simulink model "SD2231_Lab1_2022"  (R2020b)
settings: Solver=VariableStepAuto  StartTime=0.0  StopTime=inf  RelTol=1e-3
values from neighbouring files (symbols this model uses):
  delay = 250    [initial.m]
  K_awup = Ki_br_r/Kp_br_r    (= 10.4166666667)    [initial.m]
  K_brake = K_brake(3)    [initial.m]
  K_em = K_em(3)    [initial.m]
  Kd_br_f = 0*0.6*T_new_rl_b    (= 0)    [initial.m]
  Kd_br_r = 0.6*T_new_rl_b    (= 0.1722)    [initial.m]
  Kd_tr = 0.6*T_new    (= 0.0093)    [initial.m]
  Ki_br_f = 0.5*0.6*T_new_rl_b/L_new_rl_b^2    (= 37.3697916667)    [initial.m]
  Ki_br_r = 0.6*T_new_rl_b/L_new_rl_b^2    (= 74.7395833333)    [initial.m]
  Ki_tr = 0.6*T_new/L_new^2    (= 4.12188365651)    [initial.m]
  Kp_br_f = 1.2*T_new_rl_b/L_new_rl_b    (= 7.175)    [initial.m]
  Kp_br_r = 1.2*T_new_rl_b/L_new_rl_b    (= 7.175)    [initial.m]
  Kp_tr = 2.2*1.2*T_new/L_new    (= 0.861473684211)    [initial.m]
  N = 100    [initial.m]
  ref_br_f = 0.15    [initial.m]
  ref_br_r = 0.17-0.1    (= 0.07)    [initial.m]
  ref_tr = 0.06    [initial.m]
  step_time = 2    [initial.m]
  threshold_br_f = ref_br_f-0.05    (= 0.1)    [initial.m]
  threshold_br_r = ref_br_r-0.05    (= 0.02)    [initial.m]
  threshold_tc = ref_tr-0.02    (= 0.04)    [initial.m]
  vx_threshold = 1    [initial.m]
undefined symbols (not defined in the file or in its folder): DiscIntNeverNeededParam, Veh
libraries: CarMaker4SL x38, simulink x2, autolibmappedmotor x2
(part 3 of 4)

== system SD2231_Lab1_2022/CarMaker/Your ABS Controller/Activation Logic Br RR/Subsystem ==
  slip : Inport
  ref_slip : Inport  Port=2
  Brake Pedal : Inport  Port=3
  AdjBr RR : Scope
  PID1 : Subsystem
      settings: PortSchema="{\"entries\":[{\"content\":{\"sides\":[{\"content\":{\"connectorIds\":[\"In1\"]},\"type\":\"ConnectorPlacement.EquallySpacedRectSide\",\"uuid\":\"a0a678af-e4e1-4120-b7ef-0ef542f8e9cc\"},{\"content\":{\"connectorIds\":[\"Out1\"],\"side\":\"RIGHT\"},\"type\":\"ConnectorPlacement.EquallySpacedRectSide\",\"uuid\":\"903d0154-0882-4438-b528-a9d871d2aaef\"},{\"content\":{\"connectorIds\":[],\"side\":\"TOP\"},\"type\":\"ConnectorPlacement.EquallySpacedRectSide\",\"uuid\":\"cc0bbc94-fd35-44a3-99eb-327b952e9968\"},{\"content\":{\"connectorIds\":[\"In2\",\"In3\"],\"side\":\"BOTTOM\"},\"type\":\"ConnectorPlacement.EquallySpacedRectSide\",\"uuid\":\"05665a86-e33a-4510-a8ad-b2cae5a94577\"},{\"content\":{\"connectorIds\":[],\"side\":\"HIDDEN\"},\"type\":\"ConnectorPlacement.EquallySpacedRectSide\",\"uuid\":\"9e1bf206-7ec4-44f3-a0bc-dd9892acac44\"}]},\"type\":\"ConnectorPlacement.EquallySpacedConnector\",\"uuid\":\"274c0393-67a6-46bd-bc80-41d54c35eeb8\"}],\"packageUris\":[\"http://schema.mathworks.com/mf0/Connector/R2020b\"],\"version\":\"1.0\"}"
  Subtract : Sum  Inputs=+-
  AdjBr : Outport
  wires:
  Brake Pedal/1 -> PID1/3(Brake Pedal)
  Subtract/1 -> PID1/1(err)  "err_slip"
  ref_slip/1 -> Subtract/1
  slip/1 -> PID1/2(slip), Subtract/2
  PID1/1(AdjBrk) -> AdjBr/1, AdjBr RR/1  "AdjBr"

== system SD2231_Lab1_2022/CarMaker/Your ABS Controller/Activation Logic Br RR old 2/Controller ==
  slip : Inport
  ref_slip : Inport  Port=2
  Brake Pedal : Inport  Port=3
  AdjBrk RR : Scope
  PID : Subsystem
      settings: PortSchema="{\"entries\":[{\"content\":{\"sides\":[{\"content\":{\"connectorIds\":[\"In1\"]},\"type\":\"ConnectorPlacement.EquallySpacedRectSide\",\"uuid\":\"a0a678af-e4e1-4120-b7ef-0ef542f8e9cc\"},{\"content\":{\"connectorIds\":[\"Out1\"],\"side\":\"RIGHT\"},\"type\":\"ConnectorPlacement.EquallySpacedRectSide\",\"uuid\":\"903d0154-0882-4438-b528-a9d871d2aaef\"},{\"content\":{\"connectorIds\":[],\"side\":\"TOP\"},\"type\":\"ConnectorPlacement.EquallySpacedRectSide\",\"uuid\":\"cc0bbc94-fd35-44a3-99eb-327b952e9968\"},{\"content\":{\"connectorIds\":[\"In2\"],\"side\":\"BOTTOM\"},\"type\":\"ConnectorPlacement.EquallySpacedRectSide\",\"uuid\":\"05665a86-e33a-4510-a8ad-b2cae5a94577\"},{\"content\":{\"connectorIds\":[],\"side\":\"HIDDEN\"},\"type\":\"ConnectorPlacement.EquallySpacedRectSide\",\"uuid\":\"9e1bf206-7ec4-44f3-a0bc-dd9892acac44\"}]},\"type\":\"ConnectorPlacement.EquallySpacedConnector\",\"uuid\":\"274c0393-67a6-46bd-bc80-41d54c35eeb8\"}],\"packageUris\":[\"http://schema.mathworks.com/mf0/Connector/R2020b\"],\"version\":\"1.0\"}"
  Subtract : Sum  Inputs=+-
  err Br RR : Scope
  AdjThr : Outport
  wires:
  PID/1(AdjBrk) -> AdjBrk RR/1, AdjThr/1  "AdjTh"
  slip/1 -> Subtract/2
  ref_slip/1 -> Subtract/1
  Brake Pedal/1 -> PID/2(Brake Pedal)
  Subtract/1 -> err Br RR/1, PID/1(err)  "err_slip"

== system SD2231_Lab1_2022/CarMaker/Your ABS Controller/Activation Logic1/Subsystem ==
  slip : Inport
  ref_slip : Inport  Port=2
  PID : Subsystem
  Subtract : Sum  Inputs=+-
  AdjThr : Outport
  wires:
  PID/1(Out1) -> AdjThr/1  "AdjTh"
  Subtract/1 -> PID/1(err)  "err_slip"
  slip/1 -> Subtract/2
  ref_slip/1 -> Subtract/1

== system SD2231_Lab1_2022/CarMaker/Your ABS Controller/Activation Logic1/Subsystem1 ==
  slip : Inport
  ref_slip : Inport  Port=2
  y : Inport  Port=3
  Constant : Constant  Value=0
  PID : Subsystem
      settings: PortSchema="{\"entries\":[{\"content\":{\"sides\":[{\"content\":{\"connectorIds\":[\"In1\"]},\"type\":\"ConnectorPlacement.EquallySpacedRectSide\",\"uuid\":\"5f75fae0-be4e-4329-9d91-4f7d33fb87d9\"},{\"content\":{\"connectorIds\":[\"Out1\"],\"side\":\"RIGHT\"},\"type\":\"ConnectorPlacement.EquallySpacedRectSide\",\"uuid\":\"c361bfc5-4855-4965-a149-2e455cce300e\"},{\"content\":{\"connectorIds\":[],\"side\":\"TOP\"},\"type\":\"ConnectorPlacement.EquallySpacedRectSide\",\"uuid\":\"fade0fb3-5f05-4ac2-a1e9-f009226e3d9f\"},{\"content\":{\"connectorIds\":[\"In2\"],\"side\":\"BOTTOM\"},\"type\":\"ConnectorPlacement.EquallySpacedRectSide\",\"uuid\":\"3a93efea-c75a-4538-a3be-ea0ed2ce111d\"},{\"content\":{\"connectorIds\":[],\"side\":\"HIDDEN\"},\"type\":\"ConnectorPlacement.EquallySpacedRectSide\",\"uuid\":\"d2f329f2-1496-4710-b496-1fae21ed404d\"}]},\"type\":\"ConnectorPlacement.EquallySpacedConnector\",\"uuid\":\"49448e82-eaef-46f2-a659-58ee303f2511\"}],\"packageUris\":[\"http://schema.mathworks.com/mf0/Connector/R2020b\"],\"version\":\"1.0\"}"
  Subtract : Sum  Inputs=+-
  Switch : Switch  Criteria=u2 > Threshold  Threshold=0.5
  AdjThr : Outport
  wires:
  PID/1(Out1) -> AdjThr/1  "AdjTh"
  Subtract/1 -> Switch/1  "err_slip"
  ref_slip/1 -> Subtract/1
  slip/1 -> Subtract/2
  y/1 -> PID/2(y), Switch/2
  Switch/1 -> PID/1(err)
  Constant/1 -> Switch/3

== system SD2231_Lab1_2022/CarMaker/Your Traction Controller/Activation Logic RL tr1/If Action Subsystem ==
  Throttle : Inport
  Action Port : ActionPort
  Out1 : Outport
  wires:
  Throttle/1 -> Out1/1

== system SD2231_Lab1_2022/CarMaker/Your Traction Controller/Activation Logic RL tr1/Subsystem ==
  slip : Inport
  ref_slip : Inport  Port=2
  PID : Subsystem
  Subtract : Sum  Inputs=+-
  AdjThr : Outport
  wires:
  ref_slip/1 -> Subtract/1
  slip/1 -> Subtract/2
  Subtract/1 -> PID/1(err)  "err_slip"
  PID/1(Out1) -> AdjThr/1  "AdjTh"

== system SD2231_Lab1_2022/CarMaker/Your Traction Controller/Activation Logic RL tr1/Subsystem1 ==
  slip : Inport
  ref_slip : Inport  Port=2
  Thr : Inport  Port=3
  Action Port : ActionPort  InitializeStates=reset
  Add : Sum
  PID : Subsystem
  Scope : Scope
  Subtract : Sum  Inputs=+-
  AdjThr : Outport
  wires:
  slip/1 -> Subtract/2
  ref_slip/1 -> Subtract/1
  Subtract/1 -> PID/1(err)  "err_slip"
  PID/1(Out1) -> Add/1, Scope/1  "AdjTh"
  Add/1 -> AdjThr/1
  Thr/1 -> Add/2

== system SD2231_Lab1_2022/CarMaker/Your Traction Controller/Activation Logic RL tr2/Subsystem ==
  slip : Inport
  ref_slip : Inport  Port=2
  PID : Subsystem
  Subtract : Sum  Inputs=+-
  AdjThr : Outport
  wires:
  ref_slip/1 -> Subtract/1
  slip/1 -> Subtract/2
  Subtract/1 -> PID/1(err)  "err_slip"
  PID/1(Out1) -> AdjThr/1  "AdjTh"

== system SD2231_Lab1_2022/CarMaker/Your Traction Controller/Activation Logic RL tr2/Subsystem2 ==
  slip : Inport
  ref_slip : Inport  Port=2
  PID : Subsystem
  Scope : Scope
  Subtract : Sum  Inputs=+-
  AdjThr : Outport
  wires:
  PID/1(Out1) -> Scope/1, AdjThr/1  "AdjTh"
  Subtract/1 -> PID/1(err)  "err_slip"
  ref_slip/1 -> Subtract/1
  slip/1 -> Subtract/2

== system SD2231_Lab1_2022/CarMaker/Your Traction Controller/Activation Logic Tr RL/Subsystem ==
  slip : Inport
  ref_slip : Inport  Port=2
  <Throttle> : Inport  Port=3
  PID : Subsystem
      settings: PortSchema="{\"entries\":[{\"content\":{\"sides\":[{\"content\":{\"connectorIds\":[\"In1\"]},\"type\":\"ConnectorPlacement.EquallySpacedRectSide\",\"uuid\":\"27c74ca7-1daa-4fc0-829c-217569941054\"},{\"content\":{\"connectorIds\":[\"Out1\"],\"side\":\"RIGHT\"},\"type\":\"ConnectorPlacement.EquallySpacedRectSide\",\"uuid\":\"bade77b6-0597-4f1a-8de0-ed17ea00e333\"},{\"content\":{\"connectorIds\":[],\"side\":\"TOP\"},\"type\":\"ConnectorPlacement.EquallySpacedRectSide\",\"uuid\":\"4b619bdf-cd00-481e-98d9-26786e320dd0\"},{\"content\":{\"connectorIds\":[\"In2\",\"In3\"],\"side\":\"BOTTOM\"},\"type\":\"ConnectorPlacement.EquallySpacedRectSide\",\"uuid\":\"91517f3b-551d-4be5-b03a-3be9321d6908\"},{\"content\":{\"connectorIds\":[],\"side\":\"HIDDEN\"},\"type\":\"ConnectorPlacement.EquallySpacedRectSide\",\"uuid\":\"07589139-3665-4dc7-ae4e-788dbab128c2\"}]},\"type\":\"ConnectorPlacement.EquallySpacedConnector\",\"uuid\":\"e768313e-81de-4048-a761-0fa329904525\"}],\"packageUris\":[\"http://schema.mathworks.com/mf0/Connector/R2020b\"],\"version\":\"1.0\"}"
  Scope : Scope
  Subtract : Sum  Inputs=+-
  AdjThr : Outport
  wires:
  PID/1(AdjThr) -> AdjThr/1  "AdjTh"
  Subtract/1 -> Scope/1, PID/1(err)  "err_slip"
  slip/1 -> PID/2(slip), Subtract/2
  ref_slip/1 -> Subtract/1
  <Throttle>/1 -> PID/3(<Throttle>)

== system SD2231_Lab1_2022/CarMaker/Your Traction Controller/Activation Logic Tr RR/Controller ==
  slip : Inport
  ref_slip : Inport  Port=2
  Thr : Inport  Port=3
  AdjThr Tr RR : Scope
  MATLAB Function : MATLAB Function  TreatAsAtomicUnit=on
  PID : Subsystem
      settings: PortSchema="{\"entries\":[{\"content\":{\"sides\":[{\"content\":{\"connectorIds\":[\"In1\"]},\"type\":\"ConnectorPlacement.EquallySpacedRectSide\",\"uuid\":\"d5b4ba42-8bbc-455d-8ebe-912fe1a5c4b4\"},{\"content\":{\"connectorIds\":[\"Out1\"],\"side\":\"RIGHT\"},\"type\":\"ConnectorPlacement.EquallySpacedRectSide\",\"uuid\":\"23c8bac9-5734-4043-a20e-1b8e92118956\"},{\"content\":{\"connectorIds\":[\"In2\"],\"side\":\"TOP\"},\"type\":\"ConnectorPlacement.EquallySpacedRectSide\",\"uuid\":\"5c7d1d7e-636d-433e-8c10-d4c1c9edca3a\"},{\"content\":{\"connectorIds\":[],\"side\":\"HIDDEN\"},\"type\":\"ConnectorPlacement.EquallySpacedRectSide\",\"uuid\":\"05139430-708c-42b5-9da5-332763797e2c\"}]},\"type\":\"ConnectorPlacement.EquallySpacedConnector\",\"uuid\":\"3630f8de-e8d3-4428-bdc8-7dd499871779\"}],\"packageUris\":[\"http://schema.mathworks.com/mf0/Connector/R2020b\"],\"version\":\"1.0\"}"
  Subtract : Sum  Inputs=+-
  err Tr RR : Scope
  AdjThr : Outport
  wires:
  PID/1(Out1) -> AdjThr Tr RR/1, AdjThr/1  "AdjTh"
  Subtract/1 -> err Tr RR/1, PID/1(err)  "err_slip"
  slip/1 -> Subtract/2
  ref_slip/1 -> Subtract/1
  Thr/1 -> MATLAB Function/1(Brk)
  MATLAB Function/1(res) -> PID/2(res)

== system SD2231_Lab1_2022/CarMaker/Your Traction Controller/Activation Logic Tr RR/Subsystem ==
  slip : Inport
  ref_slip : Inport  Port=2
  <Throttle> : Inport  Port=3
  PID : Subsystem
      settings: PortSchema="{\"entries\":[{\"content\":{\"sides\":[{\"content\":{\"connectorIds\":[\"In1\"]},\"type\":\"ConnectorPlacement.EquallySpacedRectSide\",\"uuid\":\"27c74ca7-1daa-4fc0-829c-217569941054\"},{\"content\":{\"connectorIds\":[\"Out1\"],\"side\":\"RIGHT\"},\"type\":\"ConnectorPlacement.EquallySpacedRectSide\",\"uuid\":\"bade77b6-0597-4f1a-8de0-ed17ea00e333\"},{\"content\":{\"connectorIds\":[],\"side\":\"TOP\"},\"type\":\"ConnectorPlacement.EquallySpacedRectSide\",\"uuid\":\"4b619bdf-cd00-481e-98d9-26786e320dd0\"},{\"content\":{\"connectorIds\":[\"In2\",\"In3\"],\"side\":\"BOTTOM\"},\"type\":\"ConnectorPlacement.EquallySpacedRectSide\",\"uuid\":\"91517f3b-551d-4be5-b03a-3be9321d6908\"},{\"content\":{\"connectorIds\":[],\"side\":\"HIDDEN\"},\"type\":\"ConnectorPlacement.EquallySpacedRectSide\",\"uuid\":\"07589139-3665-4dc7-ae4e-788dbab128c2\"}]},\"type\":\"ConnectorPlacement.EquallySpacedConnector\",\"uuid\":\"e768313e-81de-4048-a761-0fa329904525\"}],\"packageUris\":[\"http://schema.mathworks.com/mf0/Connector/R2020b\"],\"version\":\"1.0\"}"
  Scope : Scope
  Subtract : Sum  Inputs=+-
  AdjThr : Outport
  wires:
  PID/1(AdjThr) -> AdjThr/1  "AdjTh"
  Subtract/1 -> Scope/1, PID/1(err)  "err_slip"
  slip/1 -> PID/2(slip), Subtract/2
  ref_slip/1 -> Subtract/1
  <Throttle>/1 -> PID/3(<Throttle>)

== system SD2231_Lab1_2022/CarMaker/Your Traction Controller/Activation Logic1/Subsystem ==
  slip : Inport
  ref_slip : Inport  Port=2
  PID : Subsystem
  Subtract : Sum  Inputs=+-
  AdjThr : Outport
  wires:
  PID/1(Out1) -> AdjThr/1  "AdjTh"
  Subtract/1 -> PID/1(err)  "err_slip"
  slip/1 -> Subtract/2
  ref_slip/1 -> Subtract/1

== system SD2231_Lab1_2022/CarMaker/Your observer/Slip observer/ FL slip subsys ==
  note: Traction Slip
  note: Braking Slip
  Vehicle velocity : Inport
  " Tyre radius" : Inport  Port=2
  Tyre rot vel : Inport  Port=3
  Divide : Product  Inputs=*/
  Divide1 : Product  Inputs=**
  Divide2 : Product  Inputs=*/
  Divide3 : Product  Inputs=**
  Saturation : Saturate  UpperLimit=inf  LowerLimit=0.5
  Saturation1 : Saturate  UpperLimit=inf  LowerLimit=0.5
  Scope : Scope  NumInputPorts=2
  Subtract1 : Sum  Inputs=-+
  Subtract2 : Sum  Inputs=+-
  trac_slip : Outport
  brak_slip : Outport  Port=2
  wires:
  Subtract2/1 -> Divide2/1  "r*w-vx"
  Subtract1/1 -> Divide/1  "r*w-vx"
  Divide2/1 -> Scope/2, brak_slip/1  "brak_slip"
  Divide/1 -> Scope/1, trac_slip/1  "trac_slip"
  Vehicle velocity/1 -> Saturation1/1, Subtract2/1, Subtract1/1
  Divide3/1 -> Subtract2/2  "r*w"
  Divide1/1 -> Saturation/1, Subtract1/2  "r*w"
  " Tyre radius"/1 -> Divide3/1, Divide1/1
  Tyre rot vel/1 -> Divide3/2, Divide1/2
  Saturation/1 -> Divide/2
  Saturation1/1 -> Divide2/2

== system SD2231_Lab1_2022/CarMaker/Your observer/Slip observer/ FR slip subsys ==
  note: Braking Slip
  note: Traction Slip
  Vehicle velocity : Inport
  " Tyre radius" : Inport  Port=2
  Tyre rot vel : Inport  Port=3
  Divide : Product  Inputs=*/
  Divide1 : Product  Inputs=**
  Divide2 : Product  Inputs=*/
  Divide3 : Product  Inputs=**
  Gain1 : Gain  Commented=on  Gain=-1
  Saturation : Saturate  UpperLimit=inf  LowerLimit=0.5
  Saturation1 : Saturate  UpperLimit=inf  LowerLimit=0.5
  Scope : Scope  NumInputPorts=2
  Subtract1 : Sum  Inputs=-+
  Subtract2 : Sum  Inputs=+-
  Switch4 : Switch  Commented=on  Criteria=u2 > Threshold
  trac_slip : Outport
  brak_slip : Outport  Port=2
  wires:
  Tyre rot vel/1 -> Divide1/2, Divide3/2
  " Tyre radius"/1 -> Divide1/1, Divide3/1
  Divide1/1 -> Saturation/1, Subtract1/2  "r*w"
  Gain1/1 -> Switch4/3
  Divide3/1 -> Subtract2/2  "r*w"
  Vehicle velocity/1 -> Subtract1/1, Saturation1/1, Subtract2/1
  Divide/1 -> trac_slip/1, Scope/1  "trac_slip"
  Divide2/1 -> brak_slip/1, Scope/2  "brak_slip"
  Subtract1/1 -> Divide/1  "r*w-vx"
  Subtract2/1 -> Divide2/1  "r*w-vx"
  Saturation/1 -> Divide/2
  Saturation1/1 -> Divide2/2

== system SD2231_Lab1_2022/CarMaker/Your observer/Slip observer/ RL slip subsys ==
  note: Braking Slip
  note: Traction Slip
  Vehicle velocity : Inport
  " Tyre radius" : Inport  Port=2
  Tyre rot vel : Inport  Port=3
  Divide : Product  Inputs=*/
  Divide1 : Product  Inputs=**
  Divide2 : Product  Inputs=*/
  Divide3 : Product  Inputs=**
  Gain1 : Gain  Commented=on  Gain=-1
  Saturation : Saturate  UpperLimit=inf  LowerLimit=0.5
  Saturation1 : Saturate  UpperLimit=inf  LowerLimit=0.5
  Scope : Scope  NumInputPorts=2
  Subtract1 : Sum  Inputs=-+
  Subtract2 : Sum  Inputs=+-
  Switch4 : Switch  Commented=on  Criteria=u2 > Threshold
  trac_slip : Outport
  brak_slip : Outport  Port=2
  wires:
  Tyre rot vel/1 -> Divide1/2, Divide3/2
  " Tyre radius"/1 -> Divide1/1, Divide3/1
  Divide1/1 -> Saturation/1, Subtract1/2  "r*w"
  Gain1/1 -> Switch4/3
  Divide3/1 -> Subtract2/2  "r*w"
  Vehicle velocity/1 -> Subtract1/1, Saturation1/1, Subtract2/1
  Divide/1 -> trac_slip/1, Scope/1  "trac_slip"
  Divide2/1 -> brak_slip/1, Scope/2  "brak_slip"
  Subtract1/1 -> Divide/1  "r*w-vx"
  Subtract2/1 -> Divide2/1  "r*w-vx"
  Saturation/1 -> Divide/2
  Saturation1/1 -> Divide2/2

== system SD2231_Lab1_2022/CarMaker/Your observer/Slip observer/ RR slip subsys ==
  note: Braking Slip
  note: Traction Slip
  Vehicle velocity : Inport
  " Tyre radius" : Inport  Port=2
  Tyre rot vel : Inport  Port=3
  Divide : Product  Inputs=*/
  Divide1 : Product  Inputs=**
  Divide2 : Product  Inputs=*/
  Divide3 : Product  Inputs=**
  Gain1 : Gain  Commented=on  Gain=-1
  Saturation : Saturate  UpperLimit=inf  LowerLimit=0.5
  Saturation1 : Saturate  UpperLimit=inf  LowerLimit=0.5
  Scope : Scope  NumInputPorts=2
  Subtract1 : Sum  Inputs=-+
  Subtract2 : Sum  Inputs=+-
  Switch4 : Switch  Commented=on  Criteria=u2 > Threshold
  trac_slip : Outport
  brak_slip : Outport  Port=2
  wires:
  Tyre rot vel/1 -> Divide1/2, Divide3/2
  " Tyre radius"/1 -> Divide1/1, Divide3/1
  Divide1/1 -> Saturation/1, Subtract1/2  "r*w"
  Gain1/1 -> Switch4/3
  Divide3/1 -> Subtract2/2  "r*w"
  Vehicle velocity/1 -> Subtract1/1, Saturation1/1, Subtract2/1
  Divide/1 -> trac_slip/1, Scope/1  "trac_slip"
  Divide2/1 -> brak_slip/1, Scope/2  "brak_slip"
  Subtract1/1 -> Divide/1  "r*w-vx"
  Subtract2/1 -> Divide2/1  "r*w-vx"
  Saturation/1 -> Divide/2
  Saturation1/1 -> Divide2/2

== system SD2231_Lab1_2022/CarMaker/IPG Vehicle/Brake/UserDefinedBrakingSystem/Subsystem ==
  FLBrakeAdjust : Inport
  BrakeFrcMax : Constant  Value=K_brake
  Gain : Gain  Gain=180.0/300.0  SaturateOnIntegerOverflow=on  OutDataTypeStr=Inherit: Same as input  ParamDataTypeStr=Inherit: Same as input
  Pedal Force : Product  InputSameDT=on  SaturateOnIntegerOverflow=on  OutDataTypeStr=Inherit: Same as first input
  Pedal Force1 : Product  InputSameDT=on  SaturateOnIntegerOverflow=on  OutDataTypeStr=Inherit: Same as first input
  pWB2Trq Front bias : Constant  Value=10
  FL brake force : Outport  VectorParamsAs1DForOutWhenUnconnected=off
  wires:
  Pedal Force/1 -> Gain/1
  BrakeFrcMax/1 -> Pedal Force/2
  Gain/1 -> Pedal Force1/1
  FLBrakeAdjust/1 -> Pedal Force/1
  pWB2Trq Front bias/1 -> Pedal Force1/2
  Pedal Force1/1 -> FL brake force/1

== system SD2231_Lab1_2022/CarMaker/IPG Vehicle/Brake/UserDefinedBrakingSystem/Subsystem1 ==
  FRBrakeAdjust : Inport
  BrakeFrcMax : Constant  Value=K_brake
  Gain : Gain  Gain=180.0/300.0  SaturateOnIntegerOverflow=on  OutDataTypeStr=Inherit: Same as input  ParamDataTypeStr=Inherit: Same as input
  Pedal Force : Product  InputSameDT=on  SaturateOnIntegerOverflow=on  OutDataTypeStr=Inherit: Same as first input
  Pedal Force1 : Product  InputSameDT=on  SaturateOnIntegerOverflow=on  OutDataTypeStr=Inherit: Same as first input
  pWB2Trq Front bias : Constant  Value=10
  FR brake force : Outport  VectorParamsAs1DForOutWhenUnconnected=off
  wires:
  Pedal Force/1 -> Gain/1
  BrakeFrcMax/1 -> Pedal Force/2
  Gain/1 -> Pedal Force1/1
  FRBrakeAdjust/1 -> Pedal Force/1
  pWB2Trq Front bias/1 -> Pedal Force1/2
  Pedal Force1/1 -> FR brake force/1

== system SD2231_Lab1_2022/CarMaker/IPG Vehicle/Brake/UserDefinedBrakingSystem/Subsystem2 ==
  RLBrakeAdjust : Inport
  BrakeFrcMax : Constant  Value=K_brake
  Gain : Gain  Gain=180.0/300.0  SaturateOnIntegerOverflow=on  OutDataTypeStr=Inherit: Same as input  ParamDataTypeStr=Inherit: Same as input
  Pedal Force : Product  InputSameDT=on  SaturateOnIntegerOverflow=on  OutDataTypeStr=Inherit: Same as first input
  Pedal Force1 : Product  InputSameDT=on  SaturateOnIntegerOverflow=on  OutDataTypeStr=Inherit: Same as first input
  pWB2Trq Rear bias : Constant  Value=4
  RL brake force : Outport  VectorParamsAs1DForOutWhenUnconnected=off
  wires:
  Pedal Force/1 -> Gain/1
  BrakeFrcMax/1 -> Pedal Force/2
  Gain/1 -> Pedal Force1/1
  RLBrakeAdjust/1 -> Pedal Force/1
  pWB2Trq Rear bias/1 -> Pedal Force1/2
  Pedal Force1/1 -> RL brake force/1

== system SD2231_Lab1_2022/CarMaker/IPG Vehicle/Brake/UserDefinedBrakingSystem/Subsystem3 ==
  RRBrakeAdjust : Inport
  BrakeFrcMax : Constant  Value=K_brake
  Gain : Gain  Gain=180.0/300.0  SaturateOnIntegerOverflow=on  OutDataTypeStr=Inherit: Same as input  ParamDataTypeStr=Inherit: Same as input
  Pedal Force : Product  InputSameDT=on  SaturateOnIntegerOverflow=on  OutDataTypeStr=Inherit: Same as first input
  Pedal Force1 : Product  InputSameDT=on  SaturateOnIntegerOverflow=on  OutDataTypeStr=Inherit: Same as first input
  pWB2Trq Rear bias : Constant  Value=4
  RR brake force : Outport  VectorParamsAs1DForOutWhenUnconnected=off
  wires:
  Pedal Force/1 -> Gain/1
  BrakeFrcMax/1 -> Pedal Force/2
  Gain/1 -> Pedal Force1/1
  RRBrakeAdjust/1 -> Pedal Force/1
  pWB2Trq Rear bias/1 -> Pedal Force1/2
  Pedal Force1/1 -> RR brake force/1

== system SD2231_Lab1_2022/CarMaker/IPG Vehicle/CarAndTrailer/CarAndTrailerUpd/CreateBus Brake.IF.In ==
  In : Inport
  BusCreator : BusCreator  Inputs=9
  Demux : Demux  Outputs=9
      settings: DisplayOption=none
  Out : Outport
  wires:
  Demux/9 -> BusCreator/9  "Brake IF Trq_Reg RR"
  Demux/8 -> BusCreator/8  "Brake IF Trq_Reg RL"
  Demux/7 -> BusCreator/7  "Brake IF Trq_Reg FR"
  Demux/6 -> BusCreator/6  "Brake IF Trq_Reg FL"
  Demux/5 -> BusCreator/5  "Brake IF Trq_Reg_max RR"
  Demux/4 -> BusCreator/4  "Brake IF Trq_Reg_max RL"
  Demux/3 -> BusCreator/3  "Brake IF Trq_Reg_max FR"
  Demux/2 -> BusCreator/2  "Brake IF Trq_Reg_max FL"
  Demux/1 -> BusCreator/1  "Brake IF T_env"
  BusCreator/1 -> Out/1
  In/1 -> Demux/1

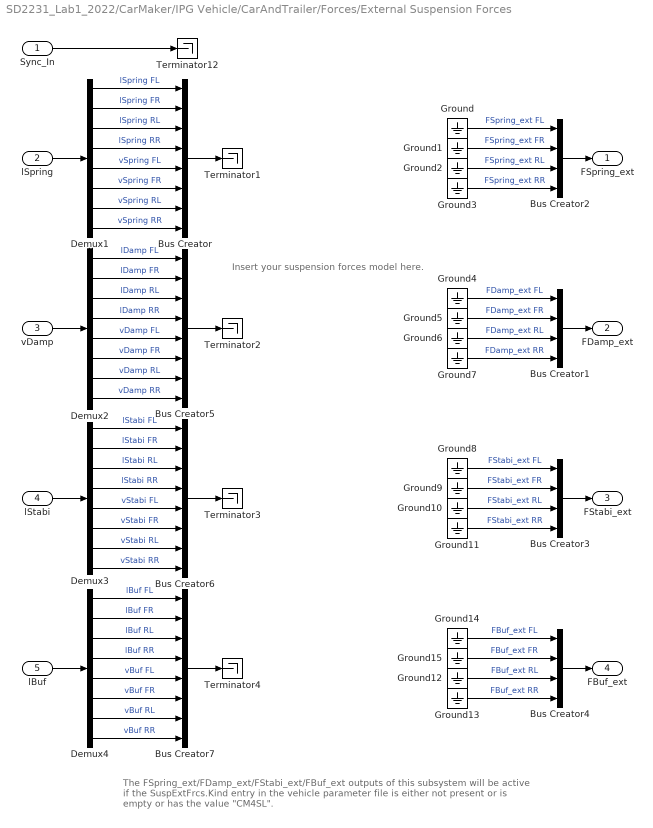
== system SD2231_Lab1_2022/CarMaker/IPG Vehicle/CarAndTrailer/Forces/External Suspension Forces ==
  note: The FSpring_ext/FDamp_ext/FStabi_ext/FBuf_ext outputs of this subsystem will be
      | active if the SuspExtFrcs.Kind entry in the vehicle parameter file
      | is either not present or is empty or has the value "CM4SL".
  note: Insert your suspension forces model here.
  Sync_In : Inport
  lSpring : Inport  Port=2
  vDamp : Inport  Port=3
  lStabi : Inport  Port=4
  lBuf : Inport  Port=5
  Bus Creator{,5..7} (4 alike) : BusCreator  Inputs=8
  Bus Creator{1..4} (4 alike) : BusCreator  Inputs=4
  Demux{1..4} (4 alike) : Demux  Outputs=8
      settings: DisplayOption=none
  Ground{,1..15} (16 alike) : Ground
  Terminator{1..4,12} (5 alike) : Terminator
  FSpring_ext : Outport
  FDamp_ext : Outport  Port=2
  FStabi_ext : Outport  Port=3
  FBuf_ext : Outport  Port=4
  wires:
  Bus Creator7/1 -> Terminator4/1
  Bus Creator6/1 -> Terminator3/1
  Bus Creator5/1 -> Terminator2/1
  Bus Creator/1 -> Terminator1/1
  Demux4/8 -> Bus Creator7/8  "vBuf RR"
  Demux4/7 -> Bus Creator7/7  "vBuf RL"
  Demux4/6 -> Bus Creator7/6  "vBuf FR"
  Demux4/5 -> Bus Creator7/5  "vBuf FL"
  Demux3/8 -> Bus Creator6/8  "vStabi RR"
  Demux3/7 -> Bus Creator6/7  "vStabi RL"
  Demux3/6 -> Bus Creator6/6  "vStabi FR"
  Demux3/5 -> Bus Creator6/5  "vStabi FL"
  Demux2/8 -> Bus Creator5/8  "vDamp RR"
  Demux2/7 -> Bus Creator5/7  "vDamp RL"
  Demux2/6 -> Bus Creator5/6  "vDamp FR"
  Demux2/5 -> Bus Creator5/5  "vDamp FL"
  Demux1/8 -> Bus Creator/8  "vSpring RR"
  Demux1/7 -> Bus Creator/7  "vSpring RL"
  Demux1/6 -> Bus Creator/6  "vSpring FR"
  Demux1/5 -> Bus Creator/5  "vSpring FL"
  Demux2/4 -> Bus Creator5/4  "lDamp RR"
  Demux2/3 -> Bus Creator5/3  "lDamp RL"
  Demux2/2 -> Bus Creator5/2  "lDamp FR"
  Demux2/1 -> Bus Creator5/1  "lDamp FL"
  Demux1/4 -> Bus Creator/4  "lSpring RR"
  Demux1/3 -> Bus Creator/3  "lSpring RL"
  Demux1/2 -> Bus Creator/2  "lSpring FR"
  Demux1/1 -> Bus Creator/1  "lSpring FL"
  Demux3/4 -> Bus Creator6/4  "lStabi RR"
  Demux3/3 -> Bus Creator6/3  "lStabi RL"
  Demux3/2 -> Bus Creator6/2  "lStabi FR"
  Demux3/1 -> Bus Creator6/1  "lStabi FL"
  lStabi/1 -> Demux3/1
  vDamp/1 -> Demux2/1
  lSpring/1 -> Demux1/1
  Demux4/4 -> Bus Creator7/4  "lBuf RR"
  Demux4/3 -> Bus Creator7/3  "lBuf RL"
  Demux4/2 -> Bus Creator7/2  "lBuf FR"
  Demux4/1 -> Bus Creator7/1  "lBuf FL"
  lBuf/1 -> Demux4/1
  Ground14/1 -> Bus Creator4/1  "FBuf_ext FL"
  Ground15/1 -> Bus Creator4/2  "FBuf_ext FR"
  Ground12/1 -> Bus Creator4/3  "FBuf_ext RL"
  Ground13/1 -> Bus Creator4/4  "FBuf_ext RR"
  Bus Creator4/1 -> FBuf_ext/1
  Sync_In/1 -> Terminator12/1
  Bus Creator2/1 -> FSpring_ext/1
  Ground/1 -> Bus Creator2/1  "FSpring_ext FL"
  Ground1/1 -> Bus Creator2/2  "FSpring_ext FR"
  Ground2/1 -> Bus Creator2/3  "FSpring_ext RL"
  Ground3/1 -> Bus Creator2/4  "FSpring_ext RR"
  Ground4/1 -> Bus Creator1/1  "FDamp_ext FL"
  Ground5/1 -> Bus Creator1/2  "FDamp_ext FR"
  Ground6/1 -> Bus Creator1/3  "FDamp_ext RL"
  Ground7/1 -> Bus Creator1/4  "FDamp_ext RR"
  Bus Creator1/1 -> FDamp_ext/1
  Ground8/1 -> Bus Creator3/1  "FStabi_ext FL"
  Ground9/1 -> Bus Creator3/2  "FStabi_ext FR"
  Ground10/1 -> Bus Creator3/3  "FStabi_ext RL"
  Ground11/1 -> Bus Creator3/4  "FStabi_ext RR"
  Bus Creator3/1 -> FStabi_ext/1

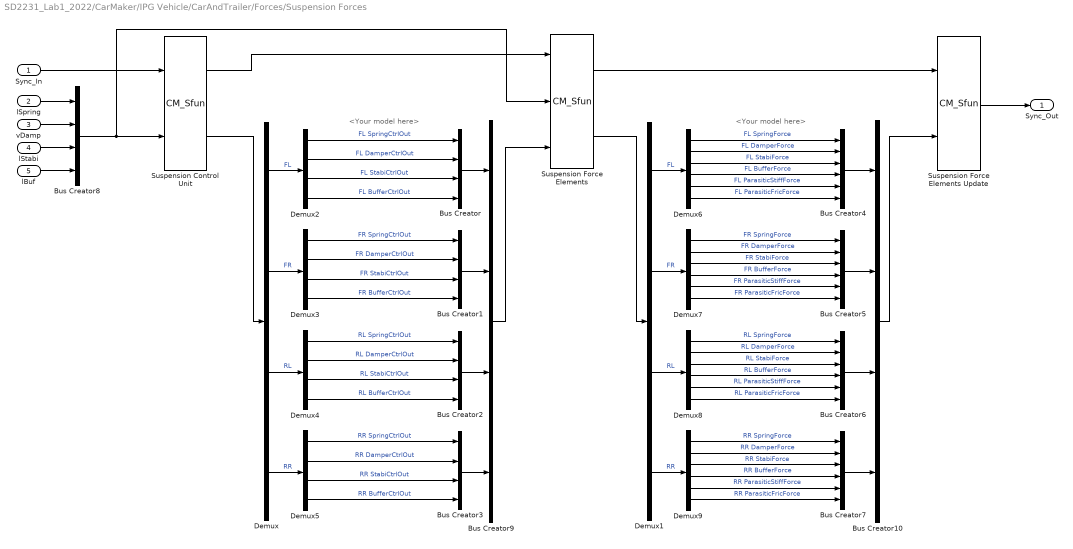
== system SD2231_Lab1_2022/CarMaker/IPG Vehicle/CarAndTrailer/Forces/Suspension Forces ==
  note: <Your model here>
  note: <Your model here>
  Sync_In : Inport
  lSpring : Inport  Port=2
  vDamp : Inport  Port=3
  lStabi : Inport  Port=4
  lBuf : Inport  Port=5
  Bus Creator{,1..3,8..10} (7 alike) : BusCreator  Inputs=4
  Bus Creator{4..7} (4 alike) : BusCreator  Inputs=6
  Demux{,1..5} (6 alike) : Demux
  Demux{6..9} (4 alike) : Demux  Outputs=6
  Suspension Control Unit : S-Function  FunctionName=CM_Sfun  Parameters='ForcesSuspControl'  SFunctionDeploymentMode=off  EnableBusSupport=off
  Suspension Force Elements : S-Function  FunctionName=CM_Sfun  Parameters='ForcesSusp'  SFunctionDeploymentMode=off  EnableBusSupport=off
  Suspension Force Elements Update : S-Function  FunctionName=CM_Sfun  Parameters='ForcesSuspUpd'  SFunctionDeploymentMode=off  EnableBusSupport=off
  Sync_Out : Outport
  wires:
  vDamp/1 -> Bus Creator8/2
  lStabi/1 -> Bus Creator8/3
  lBuf/1 -> Bus Creator8/4
  lSpring/1 -> Bus Creator8/1
  Bus Creator8/1 -> Suspension Control Unit/2, Suspension Force Elements/2
  Sync_In/1 -> Suspension Control Unit/1
  Suspension Control Unit/1 -> Suspension Force Elements/1
  Suspension Force Elements/1 -> Suspension Force Elements Update/1
  Suspension Force Elements Update/1 -> Sync_Out/1
  Bus Creator4/1 -> Bus Creator10/1
  Bus Creator5/1 -> Bus Creator10/2
  Bus Creator6/1 -> Bus Creator10/3
  Bus Creator7/1 -> Bus Creator10/4
  Demux6/1 -> Bus Creator4/1  "FL SpringForce"
  Demux9/1 -> Bus Creator7/1  "RR SpringForce"
  Demux9/2 -> Bus Creator7/2  "RR DamperForce"
  Demux9/3 -> Bus Creator7/3  "RR StabiForce"
  Demux9/4 -> Bus Creator7/4  "RR BufferForce"
  Demux9/5 -> Bus Creator7/5  "RR ParasiticStiffForce"
  Demux9/6 -> Bus Creator7/6  "RR ParasiticFricForce"
  Demux8/1 -> Bus Creator6/1  "RL SpringForce"
  Demux8/2 -> Bus Creator6/2  "RL DamperForce"
  Demux8/4 -> Bus Creator6/4  "RL BufferForce"
  Demux8/5 -> Bus Creator6/5  "RL ParasiticStiffForce"
  Demux8/6 -> Bus Creator6/6  "RL ParasiticFricForce"
  Demux8/3 -> Bus Creator6/3  "RL StabiForce"
  Demux7/1 -> Bus Creator5/1  "FR SpringForce"
  Demux7/2 -> Bus Creator5/2  "FR DamperForce"
  Demux7/3 -> Bus Creator5/3  "FR StabiForce"
  Demux7/4 -> Bus Creator5/4  "FR BufferForce"
  Demux7/5 -> Bus Creator5/5  "FR ParasiticStiffForce"
  Demux7/6 -> Bus Creator5/6  "FR ParasiticFricForce"
  Demux6/2 -> Bus Creator4/2  "FL DamperForce"
  Demux6/3 -> Bus Creator4/3  "FL StabiForce"
  Demux6/4 -> Bus Creator4/4  "FL BufferForce"
  Demux6/5 -> Bus Creator4/5  "FL ParasiticStiffForce"
  Demux6/6 -> Bus Creator4/6  "FL ParasiticFricForce"
  Bus Creator10/1 -> Suspension Force Elements Update/2
  Demux/1 -> Demux2/1  "FL"
  Bus Creator1/1 -> Bus Creator9/2
  Demux/2 -> Demux3/1  "FR"
  Bus Creator2/1 -> Bus Creator9/3
  Demux/3 -> Demux4/1  "RL"
  Bus Creator3/1 -> Bus Creator9/4
  Demux2/1 -> Bus Creator/1  "FL SpringCtrlOut"
  Demux/4 -> Demux5/1  "RR"
  Demux5/1 -> Bus Creator3/1  "RR SpringCtrlOut"
  Demux5/2 -> Bus Creator3/2  "RR DamperCtrlOut"
  Demux5/3 -> Bus Creator3/3  "RR StabiCtrlOut"
  Demux5/4 -> Bus Creator3/4  "RR BufferCtrlOut"
  Demux4/1 -> Bus Creator2/1  "RL SpringCtrlOut"
  Demux4/2 -> Bus Creator2/2  "RL DamperCtrlOut"
  Demux4/4 -> Bus Creator2/4  "RL BufferCtrlOut"
  Demux4/3 -> Bus Creator2/3  "RL StabiCtrlOut"
  Demux3/1 -> Bus Creator1/1  "FR SpringCtrlOut"
  Demux3/2 -> Bus Creator1/2  "FR DamperCtrlOut"
  Demux3/3 -> Bus Creator1/3  "FR StabiCtrlOut"
  Demux3/4 -> Bus Creator1/4  "FR BufferCtrlOut"
  Demux2/2 -> Bus Creator/2  "FL DamperCtrlOut"
  Demux2/3 -> Bus Creator/3  "FL StabiCtrlOut"
  Demux2/4 -> Bus Creator/4  "FL BufferCtrlOut"
  Suspension Control Unit/2 -> Demux/1
  Bus Creator9/1 -> Suspension Force Elements/3
  Bus Creator/1 -> Bus Creator9/1
  Suspension Force Elements/2 -> Demux1/1
  Demux1/1 -> Demux6/1  "FL"
  Demux1/2 -> Demux7/1  "FR"
  Demux1/3 -> Demux8/1  "RL"
  Demux1/4 -> Demux9/1  "RR"

== system SD2231_Lab1_2022/CarMaker/IPG Vehicle/CarAndTrailer/Forces/Tires ==
  note: The TireXX_Out signals will only be used if FileIdent is "CarMaker-Tire-CM4SL" in the tire parameter file!
      | An example parameter file can be found in Data/Tire/DT_CM4SL_UserTire.
  Sync_In : Inport
  TireFL_In : Inport  Port=2
  TireFR_In : Inport  Port=3
  TireRL_In : Inport  Port=4
  TireRR_In : Inport  Port=5
  Bus Creator{1..4} (4 alike) : BusCreator  Inputs=11
  Demux{1..3,8} (4 alike) : Demux  Outputs=7
      settings: DisplayOption=none
  TireFL : Subsystem
  TireFR : Subsystem
  TireRL : Subsystem
  TireRR : Subsystem
  TireFL_Out : Outport
  TireFR_Out : Outport  Port=2
  TireRL_Out : Outport  Port=3
  TireRR_Out : Outport  Port=4
  wires:
  Sync_In/1 -> TireRR/1(Sync_In), TireRL/1(Sync_In), TireFR/1(Sync_In), TireFL/1(Sync_In)
  Bus Creator4/1 -> TireRR_Out/1
  Bus Creator2/1 -> TireRL_Out/1
  Bus Creator1/1 -> TireFR_Out/1
  Demux3/5 -> TireRR/6(Rim_turnv)  "Tire_In Rim_turnv"
  Demux3/4 -> TireRR/5(Rim_rotv)  "Tire_In Rim_rotv"
  Demux3/1 -> TireRR/2(Load)  "Tire_In Load"
  Demux3/7 -> TireRR/8(muRoad)  "Tire_In mu"
  Demux3/6 -> TireRR/7(InclinAngle)  "Tire_In Camber"
  Demux3/2 -> TireRR/3(vxtrans)  "Tire_In vxtrans"
  Demux3/3 -> TireRR/4(vytrans)  "Tire_In vytrans"
  TireRR/11(AlignTrq) -> Bus Creator4/11  "Tire_Out AlignTrq"
  TireRR/10(RollResist) -> Bus Creator4/10  "Tire_Out RollResist"
  TireRR/9(OverturnTrq) -> Bus Creator4/9  "Tire_Out OverturnTrq"
  TireRR/8(LoadFrc) -> Bus Creator4/8  "Tire_Out LoadFrc"
  TireRR/7(SideFrc) -> Bus Creator4/7  "Tire_Out SideFrc"
  TireRR/6(LongFrc) -> Bus Creator4/6  "Tire_Out LongFrc"
  TireRR/5(vBelt) -> Bus Creator4/5  "Tire_Out vBelt"
  TireRR/4(rBelt_eff) -> Bus Creator4/4  "Tire_Out rBelt_eff"
  TireRR/3(TurnSlp) -> Bus Creator4/3  "Tire_Out TurnSlp"
  TireRR/1(Slp) -> Bus Creator4/1  "Tire_Out Slp"
  TireRR/2(Alpha) -> Bus Creator4/2  "Tire_Out Alpha"
  Demux2/5 -> TireRL/6(Rim_turnv)  "Tire_In Rim_turnv"
  Demux2/4 -> TireRL/5(Rim_rotv)  "Tire_In Rim_rotv"
  Demux2/1 -> TireRL/2(Load)  "Tire_In Load"
  Demux2/7 -> TireRL/8(muRoad)  "Tire_In mu"
  Demux2/6 -> TireRL/7(InclinAngle)  "Tire_In Camber"
  Demux2/2 -> TireRL/3(vxtrans)  "Tire_In vxtrans"
  Demux2/3 -> TireRL/4(vytrans)  "Tire_In vytrans"
  TireRL/11(AlignTrq) -> Bus Creator2/11  "Tire_Out AlignTrq"
  TireRL/10(RollResist) -> Bus Creator2/10  "Tire_Out RollResist"
  TireRL/9(OverturnTrq) -> Bus Creator2/9  "Tire_Out OverturnTrq"
  TireRL/8(LoadFrc) -> Bus Creator2/8  "Tire_Out LoadFrc"
  TireRL/7(SideFrc) -> Bus Creator2/7  "Tire_Out SideFrc"
  TireRL/6(LongFrc) -> Bus Creator2/6  "Tire_Out LongFrc"
  TireRL/5(vBelt) -> Bus Creator2/5  "Tire_Out vBelt"
  TireRL/4(rBelt_eff) -> Bus Creator2/4  "Tire_Out rBelt_eff"
  TireRL/3(TurnSlp) -> Bus Creator2/3  "Tire_Out TurnSlp"
  TireRL/1(Slp) -> Bus Creator2/1  "Tire_Out Slp"
  TireRL/2(Alpha) -> Bus Creator2/2  "Tire_Out Alpha"
  Demux1/5 -> TireFR/6(Rim_turnv)  "Tire_In Rim_turnv"
  Demux1/4 -> TireFR/5(Rim_rotv)  "Tire_In Rim_rotv"
  Demux1/1 -> TireFR/2(Load)  "Tire_In Load"
  Demux1/7 -> TireFR/8(muRoad)  "Tire_In mu"
  Demux1/6 -> TireFR/7(InclinAngle)  "Tire_In Camber"
  Demux1/2 -> TireFR/3(vxtrans)  "Tire_In vxtrans"
  Demux1/3 -> TireFR/4(vytrans)  "Tire_In vytrans"
  TireFR/11(AlignTrq) -> Bus Creator1/11  "Tire_Out AlignTrq"
  TireFR/10(RollResist) -> Bus Creator1/10  "Tire_Out RollResist"
  TireFR/9(OverturnTrq) -> Bus Creator1/9  "Tire_Out OverturnTrq"
  TireFR/8(LoadFrc) -> Bus Creator1/8  "Tire_Out LoadFrc"
  TireFR/7(SideFrc) -> Bus Creator1/7  "Tire_Out SideFrc"
  TireFR/6(LongFrc) -> Bus Creator1/6  "Tire_Out LongFrc"
  TireFR/5(vBelt) -> Bus Creator1/5  "Tire_Out vBelt"
  TireFR/4(rBelt_eff) -> Bus Creator1/4  "Tire_Out rBelt_eff"
  TireFR/3(TurnSlp) -> Bus Creator1/3  "Tire_Out TurnSlp"
  TireFR/1(Slp) -> Bus Creator1/1  "Tire_Out Slp"
  TireFR/2(Alpha) -> Bus Creator1/2  "Tire_Out Alpha"
  Demux8/5 -> TireFL/6(Rim_turnv)  "Tire_In Rim_turnv"
  Demux8/4 -> TireFL/5(Rim_rotv)  "Tire_In Rim_rotv"
  TireFL_In/1 -> Demux8/1
  Demux8/1 -> TireFL/2(Load)  "Tire_In Load"
  Demux8/7 -> TireFL/8(muRoad)  "Tire_In mu"
  Demux8/6 -> TireFL/7(InclinAngle)  "Tire_In Camber"
  Demux8/2 -> TireFL/3(vxtrans)  "Tire_In vxtrans"
  Demux8/3 -> TireFL/4(vytrans)  "Tire_In vytrans"
  TireFL/11(AlignTrq) -> Bus Creator3/11  "Tire_Out AlignTrq"
  TireFL/10(RollResist) -> Bus Creator3/10  "Tire_Out RollResist"
  TireFL/9(OverturnTrq) -> Bus Creator3/9  "Tire_Out OverturnTrq"
  TireFL/8(LoadFrc) -> Bus Creator3/8  "Tire_Out LoadFrc"
  TireFL/7(SideFrc) -> Bus Creator3/7  "Tire_Out SideFrc"
  TireFL/6(LongFrc) -> Bus Creator3/6  "Tire_Out LongFrc"
  TireFL/5(vBelt) -> Bus Creator3/5  "Tire_Out vBelt"
  TireFL/4(rBelt_eff) -> Bus Creator3/4  "Tire_Out rBelt_eff"
  TireFL/3(TurnSlp) -> Bus Creator3/3  "Tire_Out TurnSlp"
  TireFL/1(Slp) -> Bus Creator3/1  "Tire_Out Slp"
  TireFL/2(Alpha) -> Bus Creator3/2  "Tire_Out Alpha"
  Bus Creator3/1 -> TireFL_Out/1
  TireFR_In/1 -> Demux1/1
  TireRL_In/1 -> Demux2/1
  TireRR_In/1 -> Demux3/1

== system SD2231_Lab1_2022/CarMaker/IPG Vehicle/CarAndTrailer/Forces/Vehicle Forces ==
  Sync_In : Inport
  Bus Creator1 : BusCreator  Inputs=12
  Bus Creator8 : BusCreator  Inputs=16
  BusCreator1 : BusCreator  Inputs=4
  BusCreator2 : BusCreator  Inputs=9
  Demux : Demux  Outputs=16
      settings: DisplayOption=none
  Demux1 : Demux  Outputs=12
      settings: DisplayOption=none
  Demux2 : Demux  Outputs=13
      settings: DisplayOption=none
  Forces : S-Function  FunctionName=CM_Sfun  Parameters='Forces'  SFunctionDeploymentMode=off  EnableBusSupport=off
  Terminator : Terminator
  Sync_Out : Outport
  Car.Virtual : Outport  Port=2
  Car.Aero : Outport  Port=3
  Car.Load : Outport  Port=4
  wires:
  BusCreator1/1 -> Terminator/1  "Aero IF (in)"
  Demux2/13 -> BusCreator2/9  "car Aero Trq_1 z"
  Demux2/12 -> BusCreator2/8  "car Aero Trq_1 y"
  Demux2/11 -> BusCreator2/7  "car Aero Trq_1 x"
  Demux2/10 -> BusCreator2/6  "car Aero Frc_1 z"
  Demux2/9 -> BusCreator2/5  "car Aero Frc_1 y"
  Demux2/8 -> BusCreator2/4  "car Aero Frc_1 x"
  Demux2/7 -> BusCreator2/3  "car Aero PoA_1 z"
  Demux2/6 -> BusCreator2/2  "car Aero PoA_1 y"
  Demux2/5 -> BusCreator2/1  "car Aero PoA_1 x"
  Demux2/4 -> BusCreator1/4  "car Aero tau_1"
  Demux2/3 -> BusCreator1/3  "car Aero ApproachVel_1 z"
  Demux2/2 -> BusCreator1/2  "car Aero ApproachVel_1 y"
  Demux2/1 -> BusCreator1/1  "car Aero ApproachVel_1 x"
  Demux/16 -> Bus Creator8/16  "Car Load_3 tz"
  Demux/15 -> Bus Creator8/15  "Car Load_3 ty"
  Demux/14 -> Bus Creator8/14  "Car Load_3 tx"
  Demux/13 -> Bus Creator8/13  "Car Load_3 mass"
  Demux1/12 -> Bus Creator1/12  "Car Virtual Trq_0 z"
  Demux1/11 -> Bus Creator1/11  "Car Virtual Trq_0 y"
  Demux1/10 -> Bus Creator1/10  "Car Virtual Trq_0 x"
  Demux1/9 -> Bus Creator1/9  "Car Virtual Trq_1 z"
  Demux1/8 -> Bus Creator1/8  "Car Virtual Trq_1 y"
  Demux1/7 -> Bus Creator1/7  "Car Virtual Trq_1 x"
  Demux1/6 -> Bus Creator1/6  "Car Virtual Frc_0 z"
  Demux1/5 -> Bus Creator1/5  "Car Virtual Frc_0 y"
  Demux1/4 -> Bus Creator1/4  "Car Virtual Frc_0 x"
  Sync_In/1 -> Forces/1
  Forces/1 -> Sync_Out/1
  BusCreator2/1 -> Car.Aero/1
  Demux1/1 -> Bus Creator1/1  "Car Virtual Frc_1 x"
  Demux1/2 -> Bus Creator1/2  "Car Virtual Frc_1 y"
  Demux1/3 -> Bus Creator1/3  "Car Virtual Frc_1 z"
  Forces/3 -> Demux2/1
  Forces/2 -> Demux1/1
  Bus Creator1/1 -> Car.Virtual/1
  Bus Creator8/1 -> Car.Load/1
  Demux/1 -> Bus Creator8/1  "Car Load_0 mass"
  Demux/2 -> Bus Creator8/2  "Car Load_0 tx"
  Demux/3 -> Bus Creator8/3  "Car Load_0 ty"
  Demux/4 -> Bus Creator8/4  "Car Load_0 tz"
  Demux/5 -> Bus Creator8/5  "Car Load_1 mass"
  Demux/6 -> Bus Creator8/6  "Car Load_1 tx"
  Demux/7 -> Bus Creator8/7  "Car Load_1 ty"
  Demux/8 -> Bus Creator8/8  "Car Load_1 tz"
  Demux/9 -> Bus Creator8/9  "Car Load_2 mass"
  Demux/10 -> Bus Creator8/10  "Car Load_2 tx"
  Demux/11 -> Bus Creator8/11  "Car Load_2 ty"
  Demux/12 -> Bus Creator8/12  "Car Load_2 tz"
  Forces/4 -> Demux/1

== system SD2231_Lab1_2022/CarMaker/IPG Vehicle/CarAndTrailer/Trailer/CreateBus Car.Hitch.FrcTrq ==
  In1 : Inport
  Bus Creator7 : BusCreator  Inputs=6
  Demux7 : Demux  Outputs=6
      settings: DisplayOption=none
  Out1 : Outport
  wires:
  In1/1 -> Demux7/1
  Bus Creator7/1 -> Out1/1
  Demux7/6 -> Bus Creator7/6  "Car Hitch Trq2Car z"
  Demux7/5 -> Bus Creator7/5  "Car Hitch Trq2Car y"
  Demux7/4 -> Bus Creator7/4  "Car Hitch Trq2Car x"
  Demux7/3 -> Bus Creator7/3  "Car Hitch Frc2Car z"
  Demux7/2 -> Bus Creator7/2  "Car Hitch Frc2Car y"
  Demux7/1 -> Bus Creator7/1  "Car Hitch Frc2Car x"

== system SD2231_Lab1_2022/CarMaker/IPG Vehicle/CarAndTrailer/Trailer/CreateBus Vhcl.Motion ==
  In1 : Inport
  BusCreator : BusCreator  Inputs=15
  Demux : Demux  Outputs=15
      settings: DisplayOption=none
  Out1 : Outport
  wires:
  Demux/15 -> BusCreator/15  "Vhcl YawAcc"
  Demux/14 -> BusCreator/14  "Vhcl YawVel"
  Demux/13 -> BusCreator/13  "Vhcl Yaw"
  Demux/12 -> BusCreator/12  "Vhcl PitchAcc"
  Demux/11 -> BusCreator/11  "Vhcl PitchVel"
  Demux/10 -> BusCreator/10  "Vhcl Pitch"
  Demux/9 -> BusCreator/9  "Vhcl RollAcc"
  Demux/8 -> BusCreator/8  "Vhcl RollVel"
  Demux/7 -> BusCreator/7  "Vhcl Roll"
  Demux/6 -> BusCreator/6  "Vhcl Hitch_Pos z"
  Demux/5 -> BusCreator/5  "Vhcl Hitch_Pos y"
  Demux/4 -> BusCreator/4  "Vhcl Hitch_Pos x"
  Demux/3 -> BusCreator/3  "Vhcl sRoad"
  Demux/2 -> BusCreator/2  "Vhcl Distance"
  Demux/1 -> BusCreator/1  "Vhcl v"
  In1/1 -> Demux/1
  BusCreator/1 -> Out1/1

== system SD2231_Lab1_2022/CarMaker/IPG Vehicle/CarAndTrailer/Trailer/CreateBus Vhcl.PoI ==
  In1 : Inport
  Bus Creator3 : BusCreator  Inputs=18
  Demux3 : Demux  Outputs=18
      settings: DisplayOption=none
  Out1 : Outport
  wires:
  Demux3/18 -> Bus Creator3/18  "Vhcl PoI_GCS Elev"
  Demux3/17 -> Bus Creator3/17  "Vhcl PoI_GCS Lat"
  Demux3/16 -> Bus Creator3/16  "Vhcl PoI_GCS Long"
  Demux3/15 -> Bus Creator3/15  "Vhcl PoI_Acc_1 z"
  Demux3/14 -> Bus Creator3/14  "Vhcl PoI_Acc_1 y"
  Demux3/13 -> Bus Creator3/13  "Vhcl PoI_Acc_1 x"
  Demux3/12 -> Bus Creator3/12  "Vhcl PoI_Vel_1 z"
  Demux3/11 -> Bus Creator3/11  "Vhcl PoI_Vel_1 y"
  Demux3/10 -> Bus Creator3/10  "Vhcl PoI_Vel_1 x"
  Demux3/9 -> Bus Creator3/9  "Vhcl PoI_Acc z"
  Demux3/8 -> Bus Creator3/8  "Vhcl PoI_Acc y"
  Demux3/7 -> Bus Creator3/7  "Vhcl PoI_Acc x"
  Demux3/6 -> Bus Creator3/6  "Vhcl PoI_Vel z"
  Demux3/5 -> Bus Creator3/5  "Vhcl PoI_Vel y"
  Demux3/4 -> Bus Creator3/4  "Vhcl PoI_Vel x"
  Demux3/3 -> Bus Creator3/3  "Vhcl PoI_Pos z"
  Demux3/2 -> Bus Creator3/2  "Vhcl PoI_Pos y"
  In1/1 -> Demux3/1
  Bus Creator3/1 -> Out1/1
  Demux3/1 -> Bus Creator3/1  "Vhcl PoI_Pos x"

== system SD2231_Lab1_2022/CarMaker/IPG Vehicle/CarAndTrailer/Trailer/CreateBus Vhcl.Steering ==
  In1 : Inport
  Bus Creator3 : BusCreator  Inputs=4
  Demux : Demux
      settings: DisplayOption=none
  Out1 : Outport
  wires:
  Bus Creator3/1 -> Out1/1
  Demux/1 -> Bus Creator3/1  "Vhcl Steering Ang"
  Demux/3 -> Bus Creator3/3  "Vhcl Steering AngAcc"
  Demux/2 -> Bus Creator3/2  "Vhcl Steering AngVel"
  Demux/4 -> Bus Creator3/4  "Vhcl Steering Trq"
  In1/1 -> Demux/1

== system SD2231_Lab1_2022/CarMaker/IPG Vehicle/CarAndTrailer/Trailer/CreateBus Vhcl.Wheel.FL ==
  In1 : Inport
  Bus Creator3 : BusCreator  Inputs=14
  Demux3 : Demux  Outputs=14
      settings: DisplayOption=none
  Out1 : Outport
  wires:
  Demux3/14 -> Bus Creator3/14  "Vhcl Wheel FL Trq_WhlBearing"
  Demux3/13 -> Bus Creator3/13  "Vhcl Wheel FL Trq_T2W"
  Demux3/12 -> Bus Creator3/12  "Vhcl Wheel FL SideSlip"
  Demux3/11 -> Bus Creator3/11  "Vhcl Wheel FL LongSlip"
  Demux3/10 -> Bus Creator3/10  "Vhcl Wheel FL vBelt"
  Demux3/9 -> Bus Creator3/9  "Vhcl Wheel FL Fz"
  Demux3/8 -> Bus Creator3/8  "Vhcl Wheel FL Fy"
  Demux3/7 -> Bus Creator3/7  "Vhcl Wheel FL Fx"
  Demux3/6 -> Bus Creator3/6  "Vhcl Wheel FL r_zxy z"
  Demux3/5 -> Bus Creator3/5  "Vhcl Wheel FL r_zxy y"
  Demux3/4 -> Bus Creator3/4  "Vhcl Wheel FL r_zxy x"
  Demux3/3 -> Bus Creator3/3  "Vhcl Wheel FL t z"
  Demux3/2 -> Bus Creator3/2  "Vhcl Wheel FL t y"
  In1/1 -> Demux3/1
  Bus Creator3/1 -> Out1/1
  Demux3/1 -> Bus Creator3/1  "Vhcl Wheel FL t x"

== system SD2231_Lab1_2022/CarMaker/IPG Vehicle/CarAndTrailer/Trailer/CreateBus Vhcl.Wheel.FR ==
  In1 : Inport
  Bus Creator3 : BusCreator  Inputs=14
  Demux3 : Demux  Outputs=14
      settings: DisplayOption=none
  Out1 : Outport
  wires:
  Demux3/14 -> Bus Creator3/14  "Vhcl Wheel FR Trq_WhlBearing"
  Demux3/13 -> Bus Creator3/13  "Vhcl Wheel FR Trq_T2W"
  Demux3/12 -> Bus Creator3/12  "Vhcl Wheel FR SideSlip"
  Demux3/11 -> Bus Creator3/11  "Vhcl Wheel FR LongSlip"
  Demux3/10 -> Bus Creator3/10  "Vhcl Wheel FR vBelt"
  Demux3/9 -> Bus Creator3/9  "Vhcl Wheel FR Fz"
  Demux3/8 -> Bus Creator3/8  "Vhcl Wheel FR Fy"
  Demux3/7 -> Bus Creator3/7  "Vhcl Wheel FR Fx"
  Demux3/6 -> Bus Creator3/6  "Vhcl Wheel FR r_zxy z"
  Demux3/5 -> Bus Creator3/5  "Vhcl Wheel FR r_zxy y"
  Demux3/4 -> Bus Creator3/4  "Vhcl Wheel FR r_zxy x"
  Demux3/3 -> Bus Creator3/3  "Vhcl Wheel FR t z"
  Demux3/2 -> Bus Creator3/2  "Vhcl Wheel FR t y"
  In1/1 -> Demux3/1
  Bus Creator3/1 -> Out1/1
  Demux3/1 -> Bus Creator3/1  "Vhcl Wheel FR t x"

== system SD2231_Lab1_2022/CarMaker/IPG Vehicle/CarAndTrailer/Trailer/CreateBus Vhcl.Wheel.RL ==
  In1 : Inport
  Bus Creator3 : BusCreator  Inputs=14
  Demux3 : Demux  Outputs=14
      settings: DisplayOption=none
  Out1 : Outport
  wires:
  Demux3/14 -> Bus Creator3/14  "Vhcl Wheel RL Trq_WhlBearing"
  Demux3/13 -> Bus Creator3/13  "Vhcl Wheel RL Trq_T2W"
  Demux3/12 -> Bus Creator3/12  "Vhcl Wheel RL SideSlip"
  Demux3/11 -> Bus Creator3/11  "Vhcl Wheel RL LongSlip"
  Demux3/10 -> Bus Creator3/10  "Vhcl Wheel RL vBelt"
  Demux3/9 -> Bus Creator3/9  "Vhcl Wheel RL Fz"
  Demux3/8 -> Bus Creator3/8  "Vhcl Wheel RL Fy"
  Demux3/7 -> Bus Creator3/7  "Vhcl Wheel RL Fx"
  Demux3/6 -> Bus Creator3/6  "Vhcl Wheel RL r_zxy z"
  Demux3/5 -> Bus Creator3/5  "Vhcl Wheel RL r_zxy y"
  Demux3/4 -> Bus Creator3/4  "Vhcl Wheel RL r_zxy x"
  Demux3/3 -> Bus Creator3/3  "Vhcl Wheel RL t z"
  Demux3/2 -> Bus Creator3/2  "Vhcl Wheel RL t y"
  In1/1 -> Demux3/1
  Bus Creator3/1 -> Out1/1
  Demux3/1 -> Bus Creator3/1  "Vhcl Wheel RL t x"

== system SD2231_Lab1_2022/CarMaker/IPG Vehicle/CarAndTrailer/Trailer/CreateBus Vhcl.Wheel.RR ==
  In1 : Inport
  Bus Creator3 : BusCreator  Inputs=14
  Demux3 : Demux  Outputs=14
      settings: DisplayOption=none
  Out1 : Outport
  wires:
  Demux3/14 -> Bus Creator3/14  "Vhcl Wheel RR Trq_WhlBearing"
  Demux3/13 -> Bus Creator3/13  "Vhcl Wheel RR Trq_T2W"
  Demux3/12 -> Bus Creator3/12  "Vhcl Wheel RR SideSlip"
  Demux3/11 -> Bus Creator3/11  "Vhcl Wheel RR LongSlip"
  Demux3/10 -> Bus Creator3/10  "Vhcl Wheel RR vBelt"
  Demux3/9 -> Bus Creator3/9  "Vhcl Wheel RR Fz"
  Demux3/8 -> Bus Creator3/8  "Vhcl Wheel RR Fy"
  Demux3/7 -> Bus Creator3/7  "Vhcl Wheel RR Fx"
  Demux3/6 -> Bus Creator3/6  "Vhcl Wheel RR r_zxy z"
  Demux3/5 -> Bus Creator3/5  "Vhcl Wheel RR r_zxy y"
  Demux3/4 -> Bus Creator3/4  "Vhcl Wheel RR r_zxy x"
  Demux3/3 -> Bus Creator3/3  "Vhcl Wheel RR t z"
  Demux3/2 -> Bus Creator3/2  "Vhcl Wheel RR t y"
  In1/1 -> Demux3/1
  Bus Creator3/1 -> Out1/1
  Demux3/1 -> Bus Creator3/1  "Vhcl Wheel RR t x"

== system SD2231_Lab1_2022/CarMaker/IPG Vehicle/PowerTrain/User RearDriven PowerTrain1/LR Motor ==
  Gas : Inport
  "Motor speed " : Inport  Port=2
  Mapped Motor : autolibmappedmotor/Mapped Motor  port_config=Speed  param_by=Tabulated torque-speed envelope  w_t=[ 0 500 5000 10000 16000]  T_t=[440 440 350 300 280]  torque_max=.1  power_max=30  Tc=0.02  param_loss=Single efficiency measurement  eff=100  w_eff=375  T_eff=440  Piron=0  Pbase=0  w_eff_bp=[-8000 -4000 0 4000 8000]  T_eff_bp=[0 0.03 0.06 0.09]  Temp_eff_bp=[233.15 293.15 373.15]  losses_table=[1.49 1.67 2.21 3.10; 0.42 0.69 1.14 2.03; 0.06 0.24 0.78 1.68; 0.42 0.69 1.14 2.03; 1.49 1.67 2.21 3.10]  losses_table_3d=cat(3,1.05*[1.49 1.67 2.21 3.10; 0.42 0.69 1.14 2.03; 0.06 0.24 0.78 1.68; 0.42 0.69 1.14 2.03; 1.49 1.67 2.21 3.10],[1.49 1.67 2.21 3.10; 0.42 0.69 1.14 2.03; 0.06 0.24 0.78 1.68; 0.42 0.69 1.14 2.03; 1.49 1.67 2.21 3.10],1.03*[1.49 1.67 2.21 3.10; 0.42 0.69 1.14 2.03; 0.06 0.24 0.78 1.68; 0.42 0.69 1.14 2.03; 1.49 1.67 2.21 3.10])  efficiency_table=[95 95 95 95; 95 95 95 95; 95 95 95 95; 95 95 95 95; 95 95 95 95]  efficiency_table_3d=cat(3,90*ones(5,4),95*ones(5,4),92*ones(5,4))  J=0.002  b=1e-5  omega_o=0  T_t_extended=[280 300 350 440 440 440 350 300 280]  w_t_extended=[-16000 -10000 -5000 -500 0 500 5000 10000 16000]  KLossIron=0  KLossCopper=0  x_w_eff_vec=[-8000 -4000 0 4000 8000]  x_T_eff_vec=[-0.09 -0.06 -0.03 0 0.03 0.06 0.09]  x_tmp_eff_vec=[233.15 293.15 373.15]  x_losses_mat=[3.1 2.21 1.67 1.49 1.67 2.21 3.1;2.03 1.14 0.69 0.42 0.69 1.14 2.03;1.68 0.78 0.24 0.06 0.24 0.78 1.68;2.03 1.14 0.69 0.42 0.69 1.14 2.03;3.1 2.21 1.67 1.49 1.67 2.21 3.1]  x_losses_mat_3d=cat(3,[3.255 2.3205 1.7535 1.5645 1.7535 2.3205 3.255;2.1315 1.197 0.7245 0.441 0.7245 1.197 2.1315;1.764 0.819 0.252 0.063 0.252 0.819 1.764;2.1315 1.197 0.7245 0.441 0.7245 1.197 2.1315;3.255 2.3205 1.7535 1.5645 1.7535 2.3205 3.255],[3.1 2.21 1.67 1.49 1.67 2.21 3.1;2.03 1.14 0.69 0.42 0.69 1.14 2.03;1.68 0.78 0.24 0.06 0.24 0.78 1.68;2.03 1.14 0.69 0.42 0.69 1.14 2.03;3.1 2.21 1.67 1.49 1.67 2.21 3.1],[3.193 2.2763 1.7201 1.5347 1.7201 2.2763 3.193;2.0909 1.1742 0.7107 0.4326 0.7107 1.1742 2.0909;1.7304 0.8034 0.2472 0.0618 0.2472 0.8034 1.7304;2.0909 1.1742 0.7107 0.4326 0.7107 1.1742 2.0909;3.193 2.2763 1.7201 1.5347 1.7201 2.2763 3.193])  CalLossMapData={}  CalLossWithTempMapData={}  aMode=2  RefBlkName='autolibmappedmotor/Mapped Motor'
      settings: SourceProductBaseCode=PW
  "Max Torque from motor " : Constant  Value=K_em
  Product : Product  RndMeth=Zero
  Read CM Dict : CarMaker4SL/Read CM Dict  xname=PT.BattHV.Volt_oc  xsync=off  xstime=Continuous
  Scope : Scope
  Terminator : Terminator
  Terminator1 : Terminator
  Motor Trq : Outport  VectorParamsAs1DForOutWhenUnconnected=off
  wires:
  Mapped Motor/3 -> Motor Trq/1
  Read CM Dict/1 -> Mapped Motor/1
  Gas/1 -> Product/1
  Product/1 -> Mapped Motor/3
  "Max Torque from motor "/1 -> Product/2
  Mapped Motor/1 -> Terminator/1
  Mapped Motor/2 -> Terminator1/1
  "Motor speed "/1 -> Scope/1, Mapped Motor/2
